simulink model "li_ion_battery_sim"  (R2017a)
settings: Solver=VariableStepAuto  StartTime=0.0  StopTime=10000  RelTol=1e-3
libraries: fl_lib x6, nesl_utility x4, elec_lib x3, pe_lib x1
settings Model: Creator=manoj  LastModifiedBy=manoj

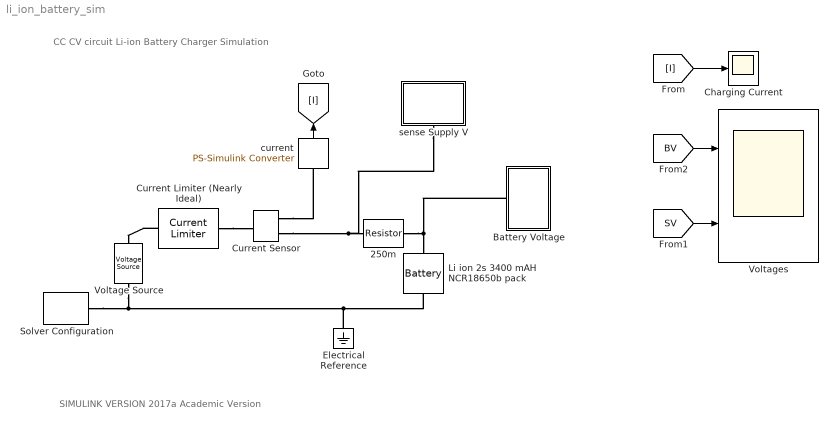
== system li_ion_battery_sim ==
  note: SIMULINK VERSION 2017a Academic Version
  note: CC CV circuit Li-ion Battery Charger Simulation
  250m : elec_lib/Passive Devices/Resistor  R=0.25 Ohm  R_tol=5  enable_R_tol=0  tol_distribution=1  nSigma=4  enable_operating_limits=0  operating_limit_action=2  max_working_voltage=100 V  power_rating=1 W  enable_faults=0  fault_action=1  R_faulted=inf Ohm  enable_temporal_fault=0  t_fault=1 s  enable_behavioral_fault=0  max_permissible_current=1 A  t_fail_on_current=1 s  noise_mode=0  sample_time=1e-3 s  repeatability=1  auto_seed=4161501170  user_seed=0  Tdevice=25 degC  alpha=3.93e-3 1/K  Tmeas=25 degC  thermal_mass=100 J/K  power_derating_T1=70 degC  power_derating_T2=155 degC  operating_temperature_range_vec=[-50.0, 150.0] degC  temperature_specify=off  temperature_priority=High  temperature=298.15 K  temperature_nominal_specify=off  temperature_nominal_unit=K  temperature_nominal_value=1
  Battery Voltage : Subsystem
  Charging Current : Scope
  Current Limiter (Nearly Ideal) : elec_lib/Semiconductor Devices/Current Limiter  iLim=1 A  vLim=0.01 V  gLim=0.01 1/Ohm  thermal_mass=100 J/K  initial_temperature=298.15 K
      settings: SourceProductName=Simscape Electronics  SourceProductBaseCode=SN
  Current Sensor : fl_lib/Electrical/Electrical Sensors/Current Sensor
  Electrical Reference : fl_lib/Electrical/Electrical Elements/Electrical Reference
  Li ion 2s 3400 mAH NCR18650b pack : pe_lib/Sources/Battery  Vnom=8.4 V  R1=0.100 Ohm  prm_AH=2  AH=3.400 hr*A  V1=8 V  AH1=2.72 hr*A  prm_R2=1  R2=2000 Ohm  prm_fade=1  N_fade=100  AH_fade=45 hr*A  R1_fade=2.02 Ohm  V1_fade=10.35 V  i_specify=off  i_priority=None  i=0 A  i_nominal_specify=off  i_nominal_unit=A  i_nominal_value=1  v_specify=on  v_priority=High  v=7 V  v_nominal_specify=off  v_nominal_unit=V  v_nominal_value=1  charge_specify=on  charge_priority=Low  charge=2 hr*A  charge_nominal_specify=off  charge_nominal_unit=hr*A  charge_nominal_value=1  num_cycles_specify=off  num_cycles_priority=High  num_cycles=0  num_cycles_nominal_specify=off  num_cycles_nominal_unit=1  num_cycles_nominal_value=1  thermal_mass=30000 J/K  Tmeas=298.15 K  Vnom_T2=12 V  R1_T2=2.2 Ohm  V1_T2=11.4 V  R2_T2=2200 Ohm  Tmeas2=273.15 K  temperature_specify=off  temperature_priority=High  temperature=298.15 K  temperature_nominal_specify=off  temperature_nominal_unit=K  temperature_nominal_value=1
      settings: SourceProductName=Simscape Power Systems  SourceProductBaseCode=PS
  Solver Configuration : nesl_utility/Solver Configuration  PhysicalDomain=network_engine_domain  SubClassName=solver  LeftPortType=input  RightPortType=generic  Accelerate=off  Tones=[]  Harmonics=[]  SimulateNoise=off  Profile=off  UseLocalSampling=off  EnableSwitchedLinearOptims=on  FrequencyDomain=off  UseCCode=off  RelTol=0.001  AbsTol=1e-06  MinStep=1e-09  ToWorkspace=off  RevertToSquareIcSolve=off  NumHomotopyIterations=100  PhasorMode=off  PhasorModeNumHarmonics=1  OverrideAbsTol=off  DoDC=off  ResidualTolerance=1e-09  UseLocalSolver=off  LocalSolverChoice=NE_BACKWARD_EULER_ADVANCER  LocalSolverSampleTime=0.001  DoFixedCost=off  MaxNonlinIter=3  MaxModeIter=2  LinearAlgebra=Sparse  DelaysMemoryBudget=1024  AutomaticFiltering=on  FilteringTimeConstant=0.001
  Voltage Source : elec_lib/Sources/Voltage Source  dc_voltage=8.4 V  ac_voltage=0 V  ac_shift=0 rad  ac_frequency=60 Hz  noise_mode=0  PSD=0 V^2/Hz  repeatability=1  auto_seed=2990441147  user_seed=0  sample_time=1e-3 s  i_specify=off  i_priority=None  i=0 A  i_nominal_specify=off  i_nominal_unit=A  i_nominal_value=1  v_specify=on  v_priority=Low  v=8.4 V  v_nominal_specify=off  v_nominal_unit=V  v_nominal_value=1
      settings: SourceProductName=Simscape Electronics  SourceProductBaseCode=SN
  Voltages : Scope  NumInputPorts=2
  current : nesl_utility/PS-Simulink Converter  PhysicalDomain=network_engine_domain  SubClassName=ps_output  LeftPortType=input  RightPortType=output  PseudoPeriodic=off  Frequencies=[]  Unit=1  AffineConversion=off
  sense Supply V : Subsystem
  wires:
  [I] -> Charging Current/1
  current/1 -> [I]
  [SV] -> Voltages/2
  [BV] -> Voltages/1
  connections:
  250m/RConn1 -- Battery Voltage/LConn1 -- Li ion 2s 3400 mAH NCR18650b pack/LConn1
  Current Sensor/RConn2 -- sense Supply V/LConn1 -- 250m/LConn1
  Current Limiter (Nearly Ideal)/LConn1 -- Voltage Source/LConn1
  Voltage Source/RConn1 -- Electrical Reference/LConn1 -- Li ion 2s 3400 mAH NCR18650b pack/RConn1 -- Solver Configuration/RConn1
  Current Limiter (Nearly Ideal)/RConn1 -- Current Sensor/LConn1
  Current Sensor/RConn1 -- current/LConn1

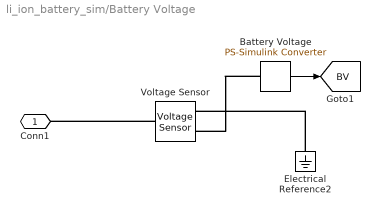
== system li_ion_battery_sim/Battery Voltage ==
  Battery Voltage : nesl_utility/PS-Simulink Converter  PhysicalDomain=network_engine_domain  SubClassName=ps_output  LeftPortType=input  RightPortType=output  PseudoPeriodic=off  Frequencies=[]  Unit=1  AffineConversion=off
  Electrical Reference2 : fl_lib/Electrical/Electrical Elements/Electrical Reference
  Voltage Sensor : fl_lib/Electrical/Electrical Sensors/Voltage Sensor
  Conn1 : PMIOPort  Port=1  Side=Left
  tag scope: BV=global
  wires:
  Battery Voltage/1 -> [BV]
  connections:
  Battery Voltage/LConn1 -- Voltage Sensor/RConn1
  Voltage Sensor/LConn1 -- Conn1/RConn1
  Electrical Reference2/LConn1 -- Voltage Sensor/RConn2

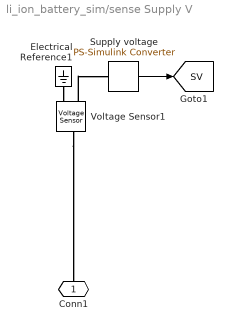
== system li_ion_battery_sim/sense Supply V ==
  Electrical Reference1 : fl_lib/Electrical/Electrical Elements/Electrical Reference
  Supply voltage : nesl_utility/PS-Simulink Converter  PhysicalDomain=network_engine_domain  SubClassName=ps_output  LeftPortType=input  RightPortType=output  PseudoPeriodic=off  Frequencies=[]  Unit=1  AffineConversion=off
  Voltage Sensor1 : fl_lib/Electrical/Electrical Sensors/Voltage Sensor
  Conn1 : PMIOPort  Port=1  Side=Left
  tag scope: SV=global
  wires:
  Supply voltage/1 -> [SV]
  connections:
  Voltage Sensor1/RConn1 -- Supply voltage/LConn1
  Voltage Sensor1/LConn1 -- Conn1/RConn1
  Electrical Reference1/LConn1 -- Voltage Sensor1/RConn2
